simulink model "ddmr_model"  (R2023b)
settings: Solver=VariableStepAuto  StartTime=0.0  StopTime=10.0  RelTol=1e-3
values from neighbouring files (symbols this model uses):
  b = constantes(7)    [calculaMatrizesModelo.m]    (also in integracaoNumerica.m = c(3); simulaModeloSimulink.m; simulaTrajetoriaSimulink.m)
  d = constantes(5)    [calculaMatrizesModelo.m]    (also in simulaModeloSimulink.m; simulaTrajetoriaSimulink.m)
  K_ce = constantes(8)    [calculaMatrizesModelo.m]    (also in simulaModeloSimulink.m; simulaTrajetoriaSimulink.m)
  K_t = constantes(9)    [calculaMatrizesModelo.m]    (also in simulaModeloSimulink.m; simulaTrajetoriaSimulink.m)
  L = constantes(2)    [calculaMatrizesModelo.m]    (also in integracaoNumerica.m = c(2); simulaModeloSimulink.m; simulaTrajetoriaSimulink.m)
  M1 = M_TRACOi(1,1)    [simulaModeloSimulink.m]    (also in simulaTrajetoriaSimulink.m)
  M2 = M_TRACOi(1,2)    [simulaModeloSimulink.m]    (also in simulaTrajetoriaSimulink.m)
  m_c = constantes(3)    [calculaMatrizesModelo.m]    (also in simulaModeloSimulink.m; simulaTrajetoriaSimulink.m)
  N = constantes(6)    [calculaMatrizesModelo.m]    (also in integracaoNumerica.m = 1; simulaModeloSimulink.m; simulaTrajetoriaSimulink.m)
  R = 0.034    [calculaErros.m]    (also in calculaMatrizesModelo.m = constantes(1); integracaoNumerica.m = c(1); plotTrajetoria.m = 0.175; simulaModeloSimulink.m = constantes(1))
  R_a = constantes(10)    [calculaMatrizesModelo.m]    (also in simulaModeloSimulink.m; simulaTrajetoriaSimulink.m)
  T = 1e-2    (= 0.01)    [otimizaControladorOnline.m]    (also in otimizaModelo.m = tempos(2)-tempos(1); otimizaModeloOffline.m; simulaModeloSimulink.m = tempo(2)-tempo(1); simulaTrajetoria.m)
settings Model: Creator=Gabriel Sousa  LastModifiedBy=Gabriel Sousa
settings DataIOCC: SaveOutput=off  DSMLogging=off  SaveTime=off
settings GRTTargetCC: CombineOutputUpdateFcns=off  MatFileLogging=off

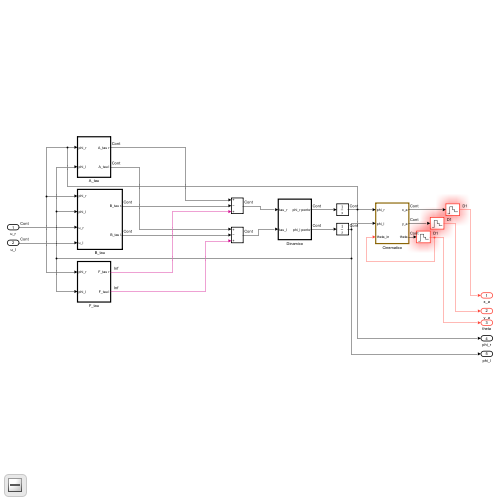
[thumbnail: Simulink's stored preview of the top-level diagram]
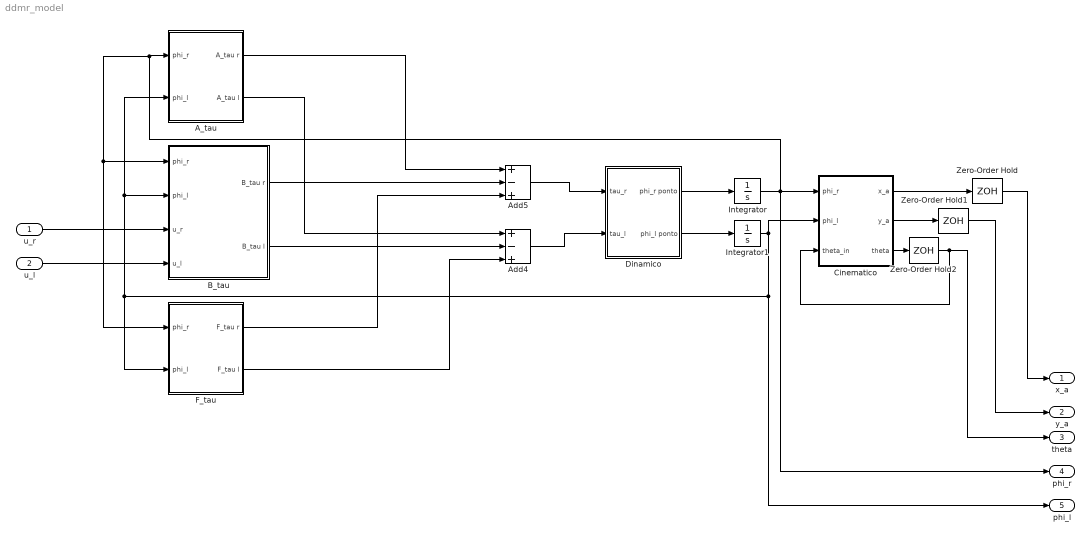
== system ddmr_model ==
  u_r : Inport
  u_l : Inport  Port=2
  A_tau : Subsystem  TreatAsAtomicUnit=on
      settings: MinAlgLoopOccurrences=on
  Add4 : Sum  Inputs=+-+
  Add5 : Sum  Inputs=+-+
  B_tau : Subsystem  TreatAsAtomicUnit=on
      settings: MinAlgLoopOccurrences=on
  Cinematico : Subsystem  TreatAsAtomicUnit=on
      settings: MinAlgLoopOccurrences=on
  Dinamico : Subsystem  TreatAsAtomicUnit=on
      settings: MinAlgLoopOccurrences=on
  F_tau : Subsystem  TreatAsAtomicUnit=on
      settings: MinAlgLoopOccurrences=on
  Integrator : Integrator
  Integrator1 : Integrator
  Zero-Order Hold : ZeroOrderHold  SampleTime=T
  Zero-Order Hold1 : ZeroOrderHold  SampleTime=T
  Zero-Order Hold2 : ZeroOrderHold  SampleTime=T
  x_a : Outport
  y_a : Outport  Port=2
  theta : Outport  Port=3
  phi_r : Outport  Port=4
  phi_l : Outport  Port=5
  wires:
  Add4/1 -> Dinamico/2(tau_l)
  B_tau/2(B_tau l) -> Add4/2
  Zero-Order Hold1/1 -> y_a/1
  Zero-Order Hold2/1 -> Cinematico/3(theta_in), theta/1
  Zero-Order Hold/1 -> x_a/1
  Add5/1 -> Dinamico/1(tau_r)
  Integrator1/1 -> B_tau/2(phi_l), A_tau/2(phi_l), F_tau/2(phi_l), phi_l/1, Cinematico/2(phi_l)
  A_tau/1(A_tau r) -> Add5/1
  B_tau/1(B_tau r) -> Add5/2
  u_r/1 -> B_tau/3(u_r)
  F_tau/2(F_tau l) -> Add4/3
  u_l/1 -> B_tau/4(u_l)
  A_tau/2(A_tau l) -> Add4/1
  Cinematico/1(x_a) -> Zero-Order Hold/1
  Dinamico/1(phi_r ponto) -> Integrator/1
  Cinematico/3(theta) -> Zero-Order Hold2/1
  Dinamico/2(phi_l ponto) -> Integrator1/1
  F_tau/1(F_tau r) -> Add5/3
  Integrator/1 -> phi_r/1, Cinematico/1(phi_r), F_tau/1(phi_r), B_tau/1(phi_r), A_tau/1(phi_r)
  Cinematico/2(y_a) -> Zero-Order Hold1/1

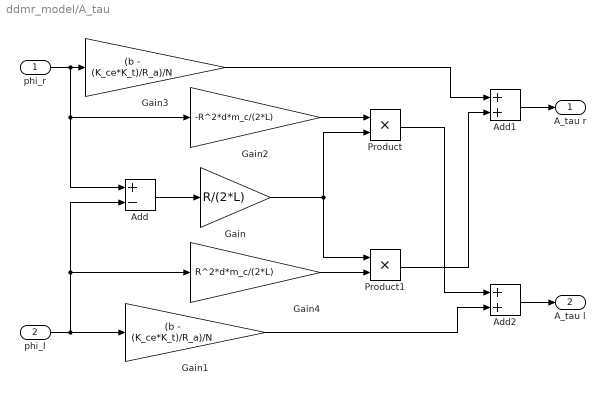
== system ddmr_model/A_tau ==
  phi_r : Inport
  phi_l : Inport  Port=2
  Add : Sum  Inputs=+-
  Add1 : Sum
  Add2 : Sum
  Gain : Gain  Gain=R/(2*L)
  Gain1 : Gain  Gain=(b - (K_ce*K_t)/R_a)/N
  Gain2 : Gain  Gain=-R^2*d*m_c/(2*L)
  Gain3 : Gain  Gain=(b - (K_ce*K_t)/R_a)/N
  Gain4 : Gain  Gain=R^2*d*m_c/(2*L)
  Product : Product
  Product1 : Product
  A_tau r : Outport
  A_tau l : Outport  Port=2
  wires:
  phi_r/1 -> Add/1, Gain2/1, Gain3/1
  Gain3/1 -> Add1/1
  Gain1/1 -> Add2/2
  phi_l/1 -> Gain1/1, Gain4/1, Add/2
  Add/1 -> Gain/1
  Gain4/1 -> Product1/2
  Gain/1 -> Product/2, Product1/1
  Gain2/1 -> Product/1
  Product1/1 -> Add1/2
  Product/1 -> Add2/1
  Add2/1 -> A_tau l/1
  Add1/1 -> A_tau r/1

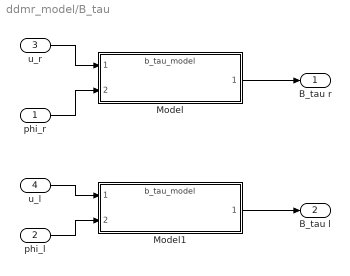
== system ddmr_model/B_tau ==
  phi_r : Inport
  phi_l : Inport  Port=2
  u_r : Inport  Port=3
  u_l : Inport  Port=4
  Model : ModelReference  ModelNameDialog=b_tau_model.slx  SimulationMode=Normal  ModelReferenceVersion=1.1
  Model1 : ModelReference  ModelNameDialog=b_tau_model.slx  SimulationMode=Normal  ModelReferenceVersion=1.1
  B_tau r : Outport
  B_tau l : Outport  Port=2
  wires:
  Model1/1 -> B_tau l/1
  u_r/1 -> Model/1
  phi_r/1 -> Model/2
  Model/1 -> B_tau r/1
  u_l/1 -> Model1/1
  phi_l/1 -> Model1/2

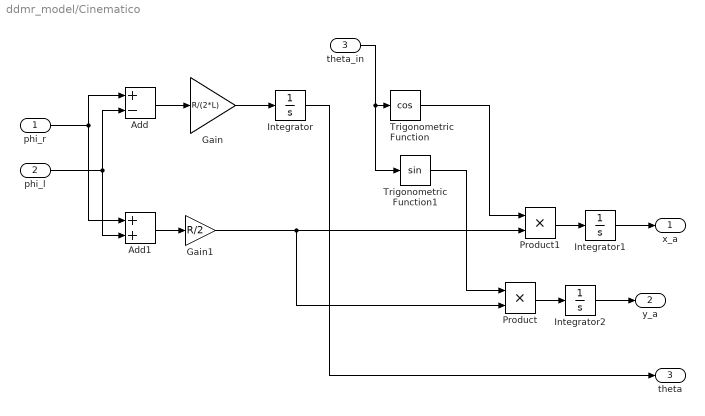
== system ddmr_model/Cinematico ==
  phi_r : Inport
  phi_l : Inport  Port=2
  theta_in : Inport  Port=3
  Add : Sum  Inputs=+-
  Add1 : Sum
  Gain : Gain  Gain=R/(2*L)
  Gain1 : Gain  Gain=R/2
  Integrator : Integrator
  Integrator1 : Integrator
  Integrator2 : Integrator
  Product : Product
  Product1 : Product
  Trigonometric Function : Trigonometry  Operator=cos  OutputSignalType=real
  Trigonometric Function1 : Trigonometry  OutputSignalType=real
  x_a : Outport  VectorParamsAs1DForOutWhenUnconnected=off
  y_a : Outport  Port=2  VectorParamsAs1DForOutWhenUnconnected=off
  theta : Outport  Port=3  VectorParamsAs1DForOutWhenUnconnected=off
  wires:
  phi_r/1 -> Add/1, Add1/1
  phi_l/1 -> Add/2, Add1/2
  Add/1 -> Gain/1
  Gain/1 -> Integrator/1
  Add1/1 -> Gain1/1
  Trigonometric Function/1 -> Product1/1
  Trigonometric Function1/1 -> Product/1
  Product/1 -> Integrator2/1
  Product1/1 -> Integrator1/1
  Integrator1/1 -> x_a/1
  Integrator2/1 -> y_a/1
  Gain1/1 -> Product1/2, Product/2
  Integrator/1 -> theta/1
  theta_in/1 -> Trigonometric Function1/1, Trigonometric Function/1

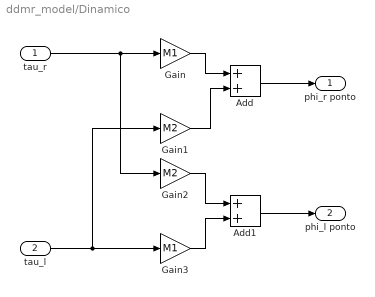
== system ddmr_model/Dinamico ==
  tau_r : Inport
  tau_l : Inport  Port=2
  Add : Sum
  Add1 : Sum
  Gain : Gain  Gain=M1
  Gain1 : Gain  Gain=M2
  Gain2 : Gain  Gain=M2
  Gain3 : Gain  Gain=M1
  phi_r ponto : Outport  VectorParamsAs1DForOutWhenUnconnected=off
  phi_l ponto : Outport  Port=2  VectorParamsAs1DForOutWhenUnconnected=off
  wires:
  Add1/1 -> phi_l ponto/1
  Gain/1 -> Add/1
  Gain1/1 -> Add/2
  Gain2/1 -> Add1/1
  Gain3/1 -> Add1/2
  tau_r/1 -> Gain/1, Gain2/1
  tau_l/1 -> Gain1/1, Gain3/1
  Add/1 -> phi_r ponto/1

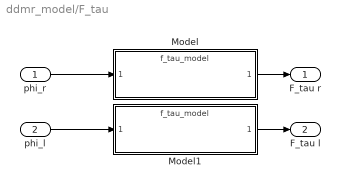
== system ddmr_model/F_tau ==
  phi_r : Inport
  phi_l : Inport  Port=2
  Model : ModelReference  ModelNameDialog=f_tau_model.slx  SimulationMode=Normal  ModelReferenceVersion=1.1
  Model1 : ModelReference  ModelNameDialog=f_tau_model.slx  SimulationMode=Normal  ModelReferenceVersion=1.1
  F_tau r : Outport
  F_tau l : Outport  Port=2
  wires:
  phi_l/1 -> Model1/1
  Model/1 -> F_tau r/1
  Model1/1 -> F_tau l/1
  phi_r/1 -> Model/1
